simulink model "LR_T_eval"  (R2021a)
settings: Solver=FixedStepAuto  StartTime=0.0  StopTime=15  FixedStep=Ts  RelTol=1e-3
undefined symbols (not defined in the file): pLander, references, u0, x0
libraries: simulink x1, mpclib x1
settings Model: Creator=The MathWorks, Inc.  LastModifiedBy=jiaya

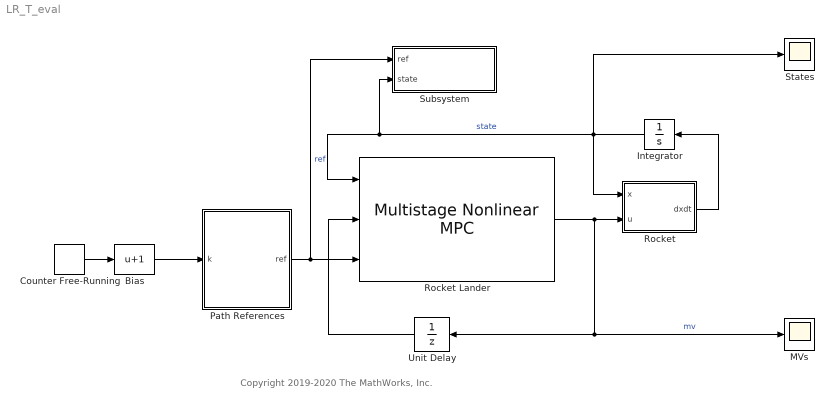
== system LR_T_eval ==
  note: Copyright 2019-2020 The MathWorks, Inc.
  Bias : Bias  Bias=1
  Counter Free-Running : simulink/Sources/Counter Free-Running  NumBits=16  tsamp=Ts
  Integrator : Integrator  InitialCondition=x0
  MVs : Scope
  Path References : MATLAB Function  TreatAsAtomicUnit=on
  Rocket : MATLAB Function  TreatAsAtomicUnit=on
  Rocket Lander : mpclib/Multistage Nonlinear MPC  SCDEnableBlockLinearizationSpecification=on  nlmpcobj=lander  UseObjectTs=on  UseMEX=off  md_enabled=off  stateparam_enabled=off  stageparam_enabled=on  cost_enabled=off  mvseq_enabled=off  stateseq_enabled=off  slack_enabled=off  status_enabled=off  mv_min=off  mv_max=off  mvrate_min=off  mvrate_max=off  state_min=off  state_max=off  terminal_state=off  nlp_initialize=off
      settings: SourceProductBaseCode=MP
  States : Scope
  Subsystem : Subsystem
  Unit Delay : UnitDelay  InitialCondition=u0  SampleTime=-1  HasFrameUpgradeWarning=on
  wires:
  Rocket Lander/1 -> Unit Delay/1, MVs/1, Rocket/2(u)  "mv"
  Rocket/1(dxdt) -> Integrator/1
  Integrator/1 -> States/1, Subsystem/2(state), Rocket Lander/1, Rocket/1(x)  "state"
  Unit Delay/1 -> Rocket Lander/2
  Path References/1(ref) -> Subsystem/1(ref), Rocket Lander/3  "ref"
  Counter Free-Running/1 -> Bias/1
  Bias/1 -> Path References/1(k)

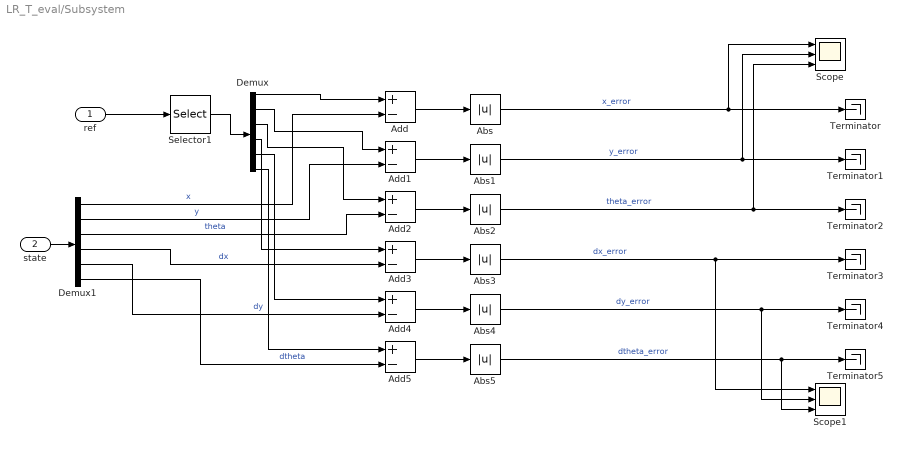
== system LR_T_eval/Subsystem ==
  ref : Inport
  state : Inport  Port=2
  Abs{,1..5} (6 alike) : Abs
  Add{,1..5} (6 alike) : Sum  Inputs=+-
  Demux : Demux  Outputs=6
  Demux1 : Demux  Outputs=6
  Scope : Scope  NumInputPorts=3
  Scope1 : Scope  NumInputPorts=3
  Selector1 : Selector  InputPortWidth=66  IndexOptions=Index vector (dialog)  Indices=[1 2 3 4 5 6]  OutputSizes=1
  Terminator{,1..5} (6 alike) : Terminator
  wires:
  Abs1/1 -> Scope/2, Terminator1/1  "y_error"
  Abs2/1 -> Scope/3, Terminator2/1  "theta_error"
  Add/1 -> Abs/1
  Selector1/1 -> Demux/1
  Add1/1 -> Abs1/1
  Demux1/2 -> Add1/2  "y"
  Demux1/1 -> Add/2  "x"
  Demux/2 -> Add1/1
  Demux1/3 -> Add2/2  "theta"
  state/1 -> Demux1/1
  Add2/1 -> Abs2/1
  Abs/1 -> Scope/1, Terminator/1  "x_error"
  Demux/1 -> Add/1
  Demux/3 -> Add2/1
  ref/1 -> Selector1/1
  Add4/1 -> Abs4/1
  Add3/1 -> Abs3/1
  Add5/1 -> Abs5/1
  Demux/4 -> Add3/1
  Demux1/4 -> Add3/2  "dx"
  Demux/5 -> Add4/1
  Demux1/5 -> Add4/2  "dy"
  Demux/6 -> Add5/1
  Demux1/6 -> Add5/2  "dtheta"
  Abs5/1 -> Scope1/3, Terminator5/1  "dtheta_error"
  Abs3/1 -> Scope1/1, Terminator3/1  "dx_error"
  Abs4/1 -> Scope1/2, Terminator4/1  "dy_error"

== matlab function LR_T_eval/Rocket ==
  data: x input; u input; dxdt output
function dxdt = fcn(x,u)
dxdt = RocketStateFcn(x,u);

== matlab function LR_T_eval/Path References ==
  data: k input; ref output; references parameter; pLander parameter
function ref = fcn(k,references,pLander)
ref = RocketLanderReferenceSignal(k,references,pLander);
